simulink model "Torque_to_Motor_Speed"  (R2020a)
settings: Solver=VariableStepAuto  StartTime=0.0  StopTime=10.0  RelTol=1e-3
settings Model: Creator=prans  LastModifiedBy=prans

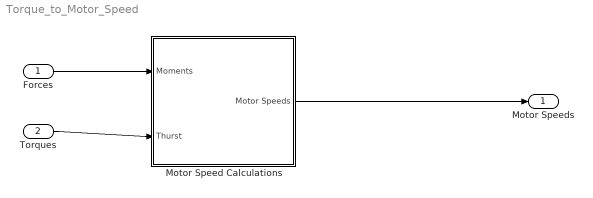
== system Torque_to_Motor_Speed ==
  Forces : Inport
  Torques : Inport  Port=2
  Motor Speed Calculations : Subsystem
  Motor Speeds : Outport
  wires:
  Forces/1 -> Motor Speed Calculations/1(Moments)
  Torques/1 -> Motor Speed Calculations/2(Thurst)
  Motor Speed Calculations/1(Motor Speeds) -> Motor Speeds/1

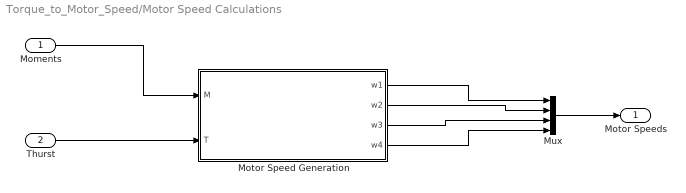
== system Torque_to_Motor_Speed/Motor Speed Calculations ==
  Moments : Inport
  Thurst : Inport  Port=2
  Motor Speed Generation : MATLAB Function  TreatAsAtomicUnit=on
  Mux : Mux
  Motor Speeds : Outport
  wires:
  Motor Speed Generation/4(w4) -> Mux/4
  Motor Speed Generation/2(w2) -> Mux/2
  Thurst/1 -> Motor Speed Generation/2(T)
  Motor Speed Generation/1(w1) -> Mux/1
  Motor Speed Generation/3(w3) -> Mux/3
  Moments/1 -> Motor Speed Generation/1(M)
  Mux/1 -> Motor Speeds/1

== matlab function Torque_to_Motor_Speed/Motor Speed Calculations/Motor Speed Generation ==
  data: M input; w1 output; w2 output; T input; w3 output; w4 output
function [w1,w2,w3,w4] = fcn(M,T)
w1 = sqrt(T/(4*k) - M(2)/(2*k*l) - m(3)/(4*b))
w2 = sqrt(T/(4/k) - M(1)/(2*k*l) + m(3)/(4*b))
w3 = sqrt(T/(4*k) + M(2)/(2*k*l) - m(3)/(4*b))
w4 = sqrt(T/(4/k) + M(1)/(2*k*l) + m(3)/(4*b))
